simulink model "test_gravity_torque_sim"  (R2021b)
settings: Solver=ode8  StartTime=0.0  StopTime=Tsim  FixedStep=0.1  RelTol=1e-3
values from neighbouring files (symbols this model uses):
  theta0 = 2*atan(sqrt((1+en)/(1-en))*tan(E/2))    [test_gravity_torque.m]
undefined symbols (not defined in the file or in its folder): i, OM, om
libraries: my_math_ops x2, kinematic_transform x1, environment x1, kinematics x1, orbit x1, dynamics x1, matrix_library x1
settings Model: Creator=Davide  LastModifiedBy=Davide

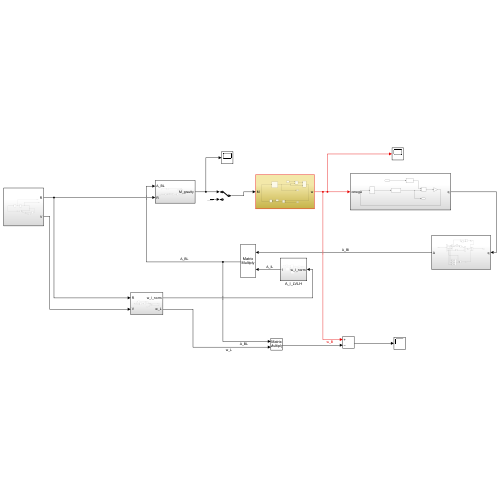
[thumbnail: Simulink's stored preview of the top-level diagram]
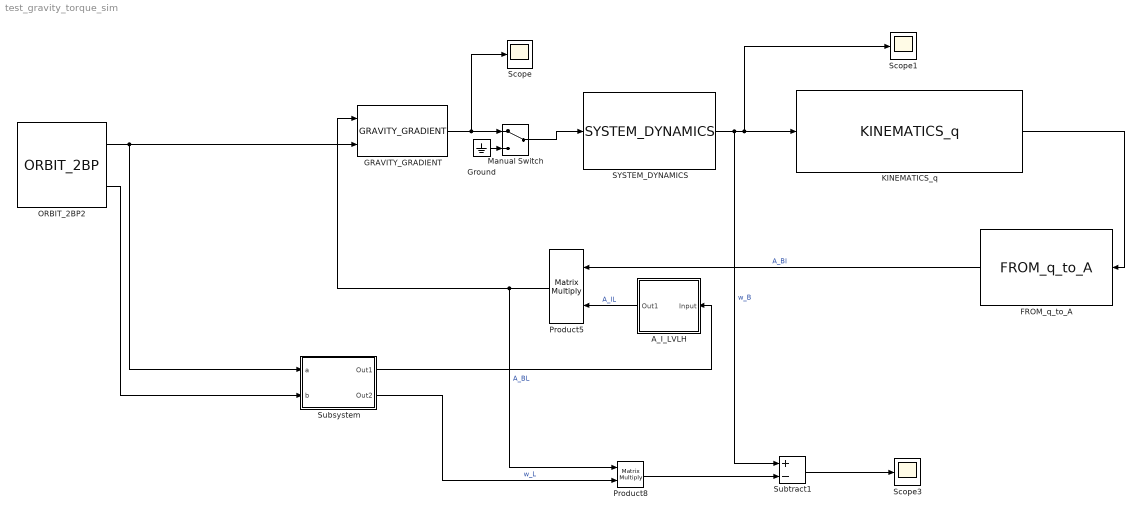
== system test_gravity_torque_sim ==
  A_I_LVLH : Subsystem
  FROM_q_to_A : kinematic_transform/FROM_q_to_A  SystemSampleTime=-1  VariantActivationTime=update diagram  Latency=0  AutoFrameSizeCalculation=off
      settings: SourceProductName=Kinematic Transformation
  GRAVITY_GRADIENT : environment/GRAVITY_GRADIENT  SystemSampleTime=-1  VariantActivationTime=update diagram  Latency=0  AutoFrameSizeCalculation=off
      settings: SourceProductName=Environment
  Ground : Ground
  KINEMATICS_q : kinematics/KINEMATICS_q  SystemSampleTime=-1  VariantActivationTime=update diagram  Latency=0  AutoFrameSizeCalculation=off
      settings: SourceProductName=Kinematics
  Manual Switch : ManualSwitch
  ORBIT_2BP2 : orbit/ORBIT_2BP  SystemSampleTime=-1  VariantActivationTime=update diagram  Latency=0  AutoFrameSizeCalculation=off
      settings: SourceProductName=Orbit
  Product5 : Product  Multiplication=Matrix(*)
  Product8 : Product  Multiplication=Matrix(*)
  SYSTEM_DYNAMICS : dynamics/SYSTEM_DYNAMICS  SystemSampleTime=-1  VariantActivationTime=update diagram  Latency=0  AutoFrameSizeCalculation=off
      settings: SourceProductName=Dynamics
  Scope : Scope
  Scope1 : Scope
  Scope3 : Scope
  Subsystem : Subsystem
  Subtract1 : Sum  Inputs=+-
  wires:
  Subtract1/1 -> Scope3/1
  Product8/1 -> Subtract1/2
  SYSTEM_DYNAMICS/1 -> Scope1/1, KINEMATICS_q/1, Subtract1/1  "w_B"
  ORBIT_2BP2/1 -> GRAVITY_GRADIENT/2, Subsystem/1(a)
  FROM_q_to_A/1 -> Product5/1  "A_BI"
  KINEMATICS_q/1 -> FROM_q_to_A/1
  A_I_LVLH/1(Out1) -> Product5/2  "A_IL"
  GRAVITY_GRADIENT/1 -> Scope/1, Manual Switch/1
  Product5/1 -> GRAVITY_GRADIENT/1, Product8/1  "A_BL"
  ORBIT_2BP2/2 -> Subsystem/2(b)
  Subsystem/1(Out1) -> A_I_LVLH/1(Input)
  Subsystem/2(Out2) -> Product8/2  "w_L"
  Manual Switch/1 -> SYSTEM_DYNAMICS/1
  Ground/1 -> Manual Switch/2

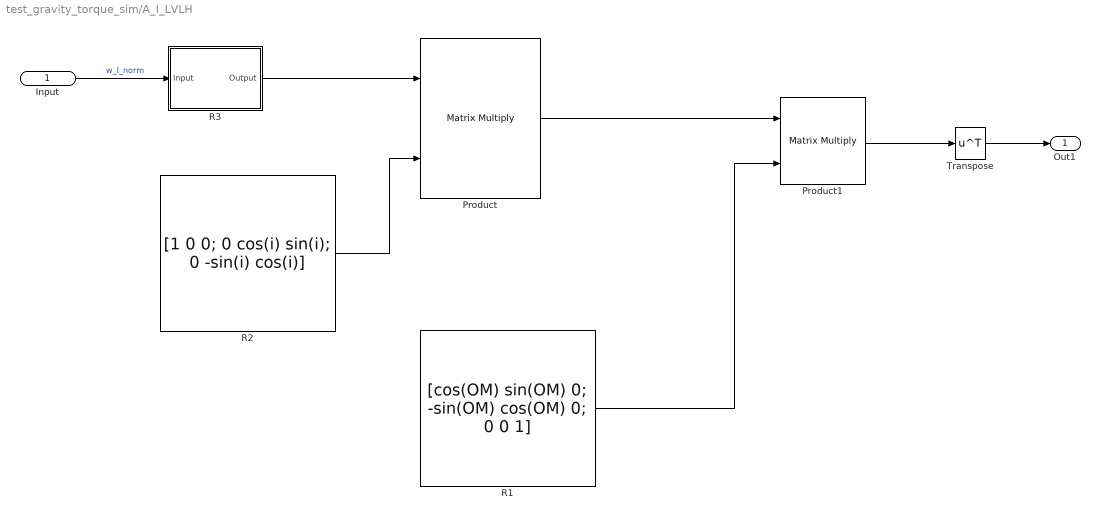
== system test_gravity_torque_sim/A_I_LVLH ==
  Input : Inport
  Product : Product  Multiplication=Matrix(*)
  Product1 : Product  Multiplication=Matrix(*)
  R1 : Constant  Value="[cos(OM)  sin(OM) 0; -sin(OM) cos(OM) 0; 0 0 1]"
  R2 : Constant  Value=[1 0 0; 0 cos(i) sin(i); 0 -sin(i) cos(i)]
  R3 : Subsystem
  Transpose : Math  Operator=transpose  SaturateOnIntegerOverflow=on
  Out1 : Outport
  wires:
  Transpose/1 -> Out1/1
  Product/1 -> Product1/1
  R2/1 -> Product/2
  Input/1 -> R3/1(Input)  "w_I_norm"
  Product1/1 -> Transpose/1
  R1/1 -> Product1/2
  R3/1(Output) -> Product/1

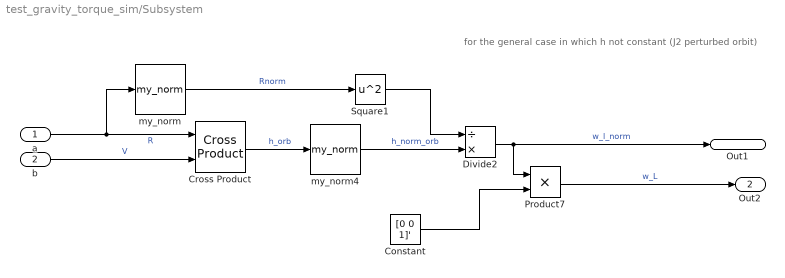
== system test_gravity_torque_sim/Subsystem ==
  note: for the general case in which h not constant (J2 perturbed orbit)
  a : Inport
  b : Inport  Port=2
  Constant : Constant  Value=[0 0 1]'
  Cross Product : matrix_library/Cross Product
      settings: SourceProductBaseCode=SL
  Divide2 : Product  Inputs=/*
  Product7 : Product
  Square1 : Math  Operator=square  SaturateOnIntegerOverflow=on
  my_norm : my_math_ops/my_norm  SystemSampleTime=-1  VariantActivationTime=update diagram  Latency=0  AutoFrameSizeCalculation=off
      settings: SourceProductName=My Mathematics Operations
  my_norm4 : my_math_ops/my_norm  SystemSampleTime=-1  VariantActivationTime=update diagram  Latency=0  AutoFrameSizeCalculation=off
      settings: SourceProductName=My Mathematics Operations
  Out1 : Outport
  Out2 : Outport  Port=2
  wires:
  my_norm/1 -> Square1/1  "Rnorm"
  Constant/1 -> Product7/2
  Square1/1 -> Divide2/1
  b/1 -> Cross Product/2  "V"
  Divide2/1 -> Out1/1, Product7/1  "w_l_norm"
  my_norm4/1 -> Divide2/2  "h_norm_orb"
  a/1 -> my_norm/1, Cross Product/1  "R"
  Cross Product/1 -> my_norm4/1  "h_orb"
  Product7/1 -> Out2/1  "w_L"

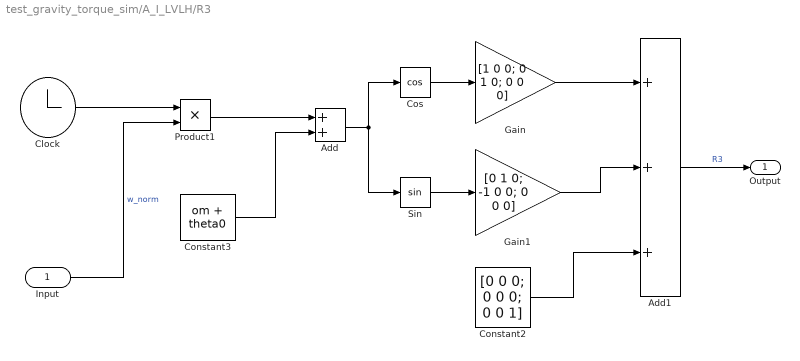
== system test_gravity_torque_sim/A_I_LVLH/R3 ==
  Input : Inport
  Add : Sum
  Add1 : Sum  Inputs=+++
  Clock : Clock
  Constant2 : Constant  Value=[0 0 0; 0 0 0; 0 0 1]
  Constant3 : Constant  Value=om + theta0
  Cos : Trigonometry  Operator=cos
  Gain : Gain  Gain=[1 0 0; 0 1 0; 0 0 0]
  Gain1 : Gain  Gain=[0 1 0; -1 0 0; 0 0 0]
  Product1 : Product
  Sin : Trigonometry
  Output : Outport
  wires:
  Clock/1 -> Product1/1
  Product1/1 -> Add/1
  Gain/1 -> Add1/1
  Add1/1 -> Output/1  "R3"
  Add/1 -> Cos/1, Sin/1
  Gain1/1 -> Add1/2
  Cos/1 -> Gain/1
  Constant3/1 -> Add/2
  Sin/1 -> Gain1/1
  Input/1 -> Product1/2  "w_norm"
  Constant2/1 -> Add1/3
